simulink model "sevietta_devel_2017j"  (R2013a)
(part 3 of 32)

      | %     if length(current_widths) ~= numios,
      | %         error('%d field names specified, but %d widths?', numios, length(current_widths));
      | %     end
      | % end
      | % total_width = 0;
      | % for ctr = 1 : length(current_widths),
      | %     total_width = total_width + current_widths(ctr);
      | % end
      | % if total_width > 32,
      | %     error('Total width must be 32 or less, set to %d.', total_width);
      | % end
      mask Callback arith_types:
      | [numios, ~, ~, ~, current_types] = swreg_maskcheck(gcb);
      | % blk = gcb;
      | % mode = get_param(blk, 'mode');
      | % current_types = eval(get_param(blk, 'arith_types'));
      | % numios = length(current_types);
      | % if (strcmp(mode, 'one value') || strcmp(mode, 'fields of equal size')) && (length(current_types) > 1),
      | %     error('Only one type may be specified for this mode.');
      | % elseif strcmp(mode, 'fields of arbitrary size')
      | %     current_names = textscan(strtrim(strrep(strrep(get_param(blk, 'names'), ']', ''), '[', '')), '%s');
      | %     current_names = current_names{1};
      | %     numios = length(current_names);
      | %     if length(current_types) ~= numios,
      | %         error('%d field names specified, but %d types?', numios, length(current_types));
      | %     end
      | % end
      | problem = 0;
      | for ctr = 1 : numios,
      |     t = current_types(ctr);
      |     if (t < 0) || (t > 2),
      |         problem = t;
      |         ctr = numios + 1;
      |     end
      | end
      | if problem ~= 0,
      |     error('Type cannot be %i, must be 0, 1 or 2.', problem);
      | end
      mask Callback bin_pts:
      | swreg_maskcheck(gcb);
      | % blk = gcb;
      | % mode = get_param(blk, 'mode');
      | % current_bins = eval(get_param(blk, 'bin_pts'));
      | % if (strcmp(mode, 'one value') || strcmp(mode, 'fields of equal size')) && (length(current_bins) > 1),
      | %     error('Only one binary pt may be specified for this mode.');
      | % elseif strcmp(mode, 'fields of arbitrary size')
      | %     current_names = textscan(strtrim(strrep(strrep(get_param(blk, 'names'), ']', ''), '[', '')), '%s');
      | %     current_names = current_names{1};
      | %     numios = length(current_names);
      | %     if length(current_bins) ~= numios,
      | %         error('%d field names specified, but %d binary pts?', numios, length(current_bins));
      | %     end
      | % end
  edge_detect1 : Subsystem  AncestorBlock=casper_library_misc/edge_detect  mask(edge_detect){edge=Rising, polarity=Active High, x_in=[0 0.08 0.08 0.16 0.16 0.24 0.24 0.32 0.32 0.4], y_in=[-1 -1  1  1  1  1  1  1  1  1], x_out=[0.6 0.68 0.68 0.76 0.76 0.84 0.84 0.92 0.92 1], y_out=[-1 -1  1  1 -1 -1 -1 -1 -1 -1]}
      mask prompts: edge "Edge Type"; polarity "Output Polarity"; x_in "Input X Positions"; y_in "Input Y Positions"; x_out "Output X Positions"; y_out "Output Y Positions"
      mask help: Output is active for one-cycle after each edge of the specified type (i.e. rising, falling or both).
      mask init:
      | edge_detect_init(gcb,...
      |     'edge',edge,...
      |     'polarity',polarity,...
      |     'x_in',x_in,...
      |     'x_out',x_out,...
      |     'y_in',y_in,...
      |     'y_out',y_out);
      | 
      | x_in_num=str2num(getfield(getfield(get_param(gcb,'UserData'),'parameters'),'x_in'));
      | x_out_num=str2num(getfield(getfield(get_param(gcb,'UserData'),'parameters'),'x_out'));
      | y_in_num=str2num(getfield(getfield(get_param(gcb,'UserData'),'parameters'),'y_in'));
      | y_out_num=str2num(getfield(getfield(get_param(gcb,'UserData'),'parameters'),'y_out'));
      settings: AttributesFormatString=|
      | rising edges
      | active high
      mask Help: Output is active for one-cycle after each edge of the specified type (i.e. rising, falling, or both).  Latency is zero.
      mask TypeOptions edge: Rising | Falling | Both
      mask TypeOptions polarity: Active High | Active Low
      mask Display:
      | plot(x_in_num,0.5+y_in_num*0.2);
      | plot(x_out_num,0.5+y_out_num*0.2);
  edge_detect2 : Subsystem  AncestorBlock=casper_library_misc/edge_detect  mask(edge_detect){edge=Rising, polarity=Active High, x_in=[0 0.08 0.08 0.16 0.16 0.24 0.24 0.32 0.32 0.4], y_in=[-1 -1  1  1  1  1  1  1  1  1], x_out=[0.6 0.68 0.68 0.76 0.76 0.84 0.84 0.92 0.92 1], y_out=[-1 -1  1  1 -1 -1 -1 -1 -1 -1]}
      mask prompts: edge "Edge Type"; polarity "Output Polarity"; x_in "Input X Positions"; y_in "Input Y Positions"; x_out "Output X Positions"; y_out "Output Y Positions"
      mask help: Output is active for one-cycle after each edge of the specified type (i.e. rising, falling or both).
      mask init: same as sevietta_devel_2017j/adc/edge_detect1
      settings: AttributesFormatString=|
      | rising edges
      | active high
      mask Help: Output is active for one-cycle after each edge of the specified type (i.e. rising, falling, or both).  Latency is zero.
      mask TypeOptions edge: Rising | Falling | Both
      mask TypeOptions polarity: Active High | Active Low
      mask Display:
      | plot(x_in_num,0.5+y_in_num*0.2);
      | plot(x_out_num,0.5+y_out_num*0.2);
  err_clear_sim{1..33} (33 alike) : Constant  Value=0
  force_sync : Subsystem  Tag=xps:sw_reg  AncestorBlock=xps_library/software_register  mask(swreg){mode=one value, io_dir=From Processor, io_delay=0, sample_period=1, names=reg, bitwidths=32, arith_types=0, bin_pts=0, sim_port=on, show_format=off}
      mask prompts: io_dir "I/O direction"; io_delay "I/O delay"; sample_period "Sample period"; names "Name:"; bitwidths "Bitwidth:"; arith_types "Type (ufix=0, fix=1, bool=2):"; bin_pts "Binary pt:"; sim_port "Provide sim input/output?"; show_format "Print format string?"
      mask init:
      | swreg_init(gcb)
      settings: AttributesFormatString=1input
      mask TypeOptions mode: one value | fields of equal size | fields of arbitrary size
      mask Callback mode: swreg_cb(gcb);
      mask TypeOptions io_dir: To Processor | From Processor
      mask Callback io_dir:
      | mask_enables = get_param(gcb, 'MaskEnables');
      | mask_names = get_param(gcb, 'MaskNames');
      | if strcmp(get_param(gcb, 'io_dir'), 'To Processor'),
      |     mask_enables{ismember(mask_names, 'sample_period')} = 'off';
      | else
      |     mask_enables{ismember(mask_names, 'sample_period')} = 'on';
      | end
      | set_param(gcb, 'MaskEnables', mask_enables);
      mask Callback bitwidths:
      | swreg_maskcheck(gcb);
      | % blk = gcb;
      | % mode = get_param(blk, 'mode');
      | % current_widths = eval(get_param(blk, 'bitwidths'));
      | % if (strcmp(mode, 'one value') || strcmp(mode, 'fields of equal size')) && (length(current_widths) > 1),
      | %     error('Only one width may be specified for this mode.');
      | % elseif strcmp(mode, 'fields of arbitrary size')
      | %     current_names = textscan(strtrim(strrep(strrep(get_param(blk, 'names'), ']', ''), '[', '')), '%s');
      | %     current_names = current_names{1};
      | %     numios = length(current_names);
      | %     if length(current_widths) ~= numios,
      | %         error('%d field names specified, but %d widths?', numios, length(current_widths));
      | %     end
      | % end
      | % total_width = 0;
      | % for ctr = 1 : length(current_widths),
      | %     total_width = total_width + current_widths(ctr);
      | % end
      | % if total_width > 32,
      | %     error('Total width must be 32 or less, set to %d.', total_width);
      | % end
      mask Callback arith_types:
      | [numios, ~, ~, ~, current_types] = swreg_maskcheck(gcb);
      | % blk = gcb;
      | % mode = get_param(blk, 'mode');
      | % current_types = eval(get_param(blk, 'arith_types'));
      | % numios = length(current_types);
      | % if (strcmp(mode, 'one value') || strcmp(mode, 'fields of equal size')) && (length(current_types) > 1),
      | %     error('Only one type may be specified for this mode.');
      | % elseif strcmp(mode, 'fields of arbitrary size')
      | %     current_names = textscan(strtrim(strrep(strrep(get_param(blk, 'names'), ']', ''), '[', '')), '%s');
      | %     current_names = current_names{1};
      | %     numios = length(current_names);
      | %     if length(current_types) ~= numios,
      | %         error('%d field names specified, but %d types?', numios, length(current_types));
      | %     end
      | % end
      | problem = 0;
      | for ctr = 1 : numios,
      |     t = current_types(ctr);
      |     if (t < 0) || (t > 2),
      |         problem = t;
      |         ctr = numios + 1;
      |     end
      | end
      | if problem ~= 0,
      |     error('Type cannot be %i, must be 0, 1 or 2.', problem);
      | end
      mask Callback bin_pts:
      | swreg_maskcheck(gcb);
      | % blk = gcb;
      | % mode = get_param(blk, 'mode');
      | % current_bins = eval(get_param(blk, 'bin_pts'));
      | % if (strcmp(mode, 'one value') || strcmp(mode, 'fields of equal size')) && (length(current_bins) > 1),
      | %     error('Only one binary pt may be specified for this mode.');
      | % elseif strcmp(mode, 'fields of arbitrary size')
      | %     current_names = textscan(strtrim(strrep(strrep(get_param(blk, 'names'), ']', ''), '[', '')), '%s');
      | %     current_names = current_names{1};
      | %     numios = length(current_names);
      | %     if length(current_bins) ~= numios,
      | %         error('%d field names specified, but %d binary pts?', numios, length(current_bins));
      | %     end
      | % end
  led_pps : xps_library/gpio  Tag=xps:gpio  io_group=ROACH2:gpio  io_dir=out  arith_type=Boolean  bitwidth=1  bin_pt=0  bit_index=0  sample_period=1  use_single_ended=off  use_ddr=off  reg_iob=on  reg_clk_phase=0  termination=None
  led_tx : xps_library/gpio  Tag=xps:gpio  io_group=ROACH2:gpio  io_dir=out  arith_type=Boolean  bitwidth=1  bin_pt=0  bit_index=1  sample_period=1  use_single_ended=off  use_ddr=off  reg_iob=on  reg_clk_phase=0  termination=None
  pipeline33 : Subsystem  AncestorBlock=casper_library_delays/pipeline  mask(pipeline){latency=1}
      mask help:
      | An explicitly laid-out delay line to avoid mapping to SRL16s
      | for use in pipelining to help achieve timing closure.
      mask init:
      | pipeline_init(gcb,'latency',latency);
      settings: AttributesFormatString=Latency = %<latency>
      mask Display:
      | port_label('input', 1, 'd');
      | port_label('output', 1, 'q');
      | disp(['Z^-', num2str(latency)]);
  pipeline34 : Subsystem  AncestorBlock=casper_library_delays/pipeline  mask(pipeline){latency=1}
      mask help:
      | An explicitly laid-out delay line to avoid mapping to SRL16s
      | for use in pipelining to help achieve timing closure.
      mask init:
      | pipeline_init(gcb,'latency',latency);
      settings: AttributesFormatString=Latency = %<latency>
      mask Display:
      | port_label('input', 1, 'd');
      | port_label('output', 1, 'q');
      | disp(['Z^-', num2str(latency)]);
  pipeline35 : Subsystem  AncestorBlock=casper_library_delays/pipeline  mask(pipeline){latency=1}
      mask help:
      | An explicitly laid-out delay line to avoid mapping to SRL16s
      | for use in pipelining to help achieve timing closure.
      mask init:
      | pipeline_init(gcb,'latency',latency);
      settings: AttributesFormatString=Latency = %<latency>
      mask Display:
      | port_label('input', 1, 'd');
      | port_label('output', 1, 'q');
      | disp(['Z^-', num2str(latency)]);
  pipeline36 : Subsystem  AncestorBlock=casper_library_delays/pipeline  mask(pipeline){latency=1}
      mask help:
      | An explicitly laid-out delay line to avoid mapping to SRL16s
      | for use in pipelining to help achieve timing closure.
      mask init:
      | pipeline_init(gcb,'latency',latency);
      settings: AttributesFormatString=Latency = %<latency>
      mask Display:
      | port_label('input', 1, 'd');
      | port_label('output', 1, 'q');
      | disp(['Z^-', num2str(latency)]);
  pipeline37 : Subsystem  AncestorBlock=casper_library_delays/pipeline  mask(pipeline){latency=1}
      mask help:
      | An explicitly laid-out delay line to avoid mapping to SRL16s
      | for use in pipelining to help achieve timing closure.
      mask init:
      | pipeline_init(gcb,'latency',latency);
      settings: AttributesFormatString=Latency = %<latency>
      mask Display:
      | port_label('input', 1, 'd');
      | port_label('output', 1, 'q');
      | disp(['Z^-', num2str(latency)]);
  pipeline38 : Subsystem  AncestorBlock=casper_library_delays/pipeline  mask(pipeline){latency=1}
      mask help:
      | An explicitly laid-out delay line to avoid mapping to SRL16s
      | for use in pipelining to help achieve timing closure.
      mask init:
      | pipeline_init(gcb,'latency',latency);
      settings: AttributesFormatString=Latency = %<latency>
      mask Display:
      | port_label('input', 1, 'd');
      | port_label('output', 1, 'q');
      | disp(['Z^-', num2str(latency)]);
  pipeline39 : Subsystem  AncestorBlock=casper_library_delays/pipeline  mask(pipeline){latency=1}
      mask help:
      | An explicitly laid-out delay line to avoid mapping to SRL16s
      | for use in pipelining to help achieve timing closure.
      mask init:
      | pipeline_init(gcb,'latency',latency);
      settings: AttributesFormatString=Latency = %<latency>
      mask Display:
      | port_label('input', 1, 'd');
      | port_label('output', 1, 'q');
      | disp(['Z^-', num2str(latency)]);
  pipeline40 : Subsystem  AncestorBlock=casper_library_delays/pipeline  mask(pipeline){latency=1}
      mask help:
      | An explicitly laid-out delay line to avoid mapping to SRL16s
      | for use in pipelining to help achieve timing closure.
      mask init:
      | pipeline_init(gcb,'latency',latency);
      settings: AttributesFormatString=Latency = %<latency>
      mask Display:
      | port_label('input', 1, 'd');
      | port_label('output', 1, 'q');
      | disp(['Z^-', num2str(latency)]);
  pipeline41 : Subsystem  AncestorBlock=casper_library_delays/pipeline  mask(pipeline){latency=1}
      mask help:
      | An explicitly laid-out delay line to avoid mapping to SRL16s
      | for use in pipelining to help achieve timing closure.
      mask init:
      | pipeline_init(gcb,'latency',latency);
      settings: AttributesFormatString=Latency = %<latency>
      mask Display:
      | port_label('input', 1, 'd');
      | port_label('output', 1, 'q');
      | disp(['Z^-', num2str(latency)]);
  pipeline42 : Subsystem  AncestorBlock=casper_library_delays/pipeline  mask(pipeline){latency=1}
      mask help:
      | An explicitly laid-out delay line to avoid mapping to SRL16s
      | for use in pipelining to help achieve timing closure.
      mask init:
      | pipeline_init(gcb,'latency',latency);
      settings: AttributesFormatString=Latency = %<latency>
      mask Display:
      | port_label('input', 1, 'd');
      | port_label('output', 1, 'q');
      | disp(['Z^-', num2str(latency)]);
  pipeline43 : Subsystem  AncestorBlock=casper_library_delays/pipeline  mask(pipeline){latency=1}
      mask help:
      | An explicitly laid-out delay line to avoid mapping to SRL16s
      | for use in pipelining to help achieve timing closure.
      mask init:
      | pipeline_init(gcb,'latency',latency);
      settings: AttributesFormatString=Latency = %<latency>
      mask Display:
      | port_label('input', 1, 'd');
      | port_label('output', 1, 'q');
      | disp(['Z^-', num2str(latency)]);
  pipeline44 : Subsystem  AncestorBlock=casper_library_delays/pipeline  mask(pipeline){latency=1}
      mask help:
      | An explicitly laid-out delay line to avoid mapping to SRL16s
      | for use in pipelining to help achieve timing closure.
      mask init:
      | pipeline_init(gcb,'latency',latency);
      settings: AttributesFormatString=Latency = %<latency>
      mask Display:
      | port_label('input', 1, 'd');
      | port_label('output', 1, 'q');
      | disp(['Z^-', num2str(latency)]);
  pipeline45 : Subsystem  AncestorBlock=casper_library_delays/pipeline  mask(pipeline){latency=1}
      mask help:
      | An explicitly laid-out delay line to avoid mapping to SRL16s
      | for use in pipelining to help achieve timing closure.
      mask init:
      | pipeline_init(gcb,'latency',latency);
      settings: AttributesFormatString=Latency = %<latency>
      mask Display:
      | port_label('input', 1, 'd');
      | port_label('output', 1, 'q');
      | disp(['Z^-', num2str(latency)]);
  pipeline46 : Subsystem  AncestorBlock=casper_library_delays/pipeline  mask(pipeline){latency=1}
      mask help:
      | An explicitly laid-out delay line to avoid mapping to SRL16s
      | for use in pipelining to help achieve timing closure.
      mask init:
      | pipeline_init(gcb,'latency',latency);
      settings: AttributesFormatString=Latency = %<latency>
      mask Display:
      | port_label('input', 1, 'd');
      | port_label('output', 1, 'q');
      | disp(['Z^-', num2str(latency)]);
  pipeline47 : Subsystem  AncestorBlock=casper_library_delays/pipeline  mask(pipeline){latency=1}
      mask help:
      | An explicitly laid-out delay line to avoid mapping to SRL16s
      | for use in pipelining to help achieve timing closure.
      mask init:
      | pipeline_init(gcb,'latency',latency);
      settings: AttributesFormatString=Latency = %<latency>
      mask Display:
      | port_label('input', 1, 'd');
      | port_label('output', 1, 'q');
      | disp(['Z^-', num2str(latency)]);
  pipeline48 : Subsystem  AncestorBlock=casper_library_delays/pipeline  mask(pipeline){latency=1}
      mask help:
      | An explicitly laid-out delay line to avoid mapping to SRL16s
      | for use in pipelining to help achieve timing closure.
      mask init:
      | pipeline_init(gcb,'latency',latency);
      settings: AttributesFormatString=Latency = %<latency>
      mask Display:
      | port_label('input', 1, 'd');
      | port_label('output', 1, 'q');
      | disp(['Z^-', num2str(latency)]);
  pipeline49 : Subsystem  AncestorBlock=casper_library_delays/pipeline  mask(pipeline){latency=1}
      mask help:
      | An explicitly laid-out delay line to avoid mapping to SRL16s
      | for use in pipelining to help achieve timing closure.
      mask init:
      | pipeline_init(gcb,'latency',latency);
      settings: AttributesFormatString=Latency = %<latency>
      mask Display:
      | port_label('input', 1, 'd');
      | port_label('output', 1, 'q');
      | disp(['Z^-', num2str(latency)]);
  pipeline50 : Subsystem  AncestorBlock=casper_library_delays/pipeline  mask(pipeline){latency=1}
      mask help:
      | An explicitly laid-out delay line to avoid mapping to SRL16s
      | for use in pipelining to help achieve timing closure.
      mask init:
      | pipeline_init(gcb,'latency',latency);
      settings: AttributesFormatString=Latency = %<latency>
      mask Display:
      | port_label('input', 1, 'd');
      | port_label('output', 1, 'q');
      | disp(['Z^-', num2str(latency)]);
  pipeline51 : Subsystem  AncestorBlock=casper_library_delays/pipeline  mask(pipeline){latency=1}
      mask help:
      | An explicitly laid-out delay line to avoid mapping to SRL16s
      | for use in pipelining to help achieve timing closure.
      mask init:
      | pipeline_init(gcb,'latency',latency);
      settings: AttributesFormatString=Latency = %<latency>
      mask Display:
      | port_label('input', 1, 'd');
      | port_label('output', 1, 'q');
      | disp(['Z^-', num2str(latency)]);
  pipeline52 : Subsystem  AncestorBlock=casper_library_delays/pipeline  mask(pipeline){latency=1}
      mask help:
      | An explicitly laid-out delay line to avoid mapping to SRL16s
      | for use in pipelining to help achieve timing closure.
      mask init:
      | pipeline_init(gcb,'latency',latency);
      settings: AttributesFormatString=Latency = %<latency>
      mask Display:
      | port_label('input', 1, 'd');
      | port_label('output', 1, 'q');
      | disp(['Z^-', num2str(latency)]);
  pipeline53 : Subsystem  AncestorBlock=casper_library_delays/pipeline  mask(pipeline){latency=1}
      mask help:
      | An explicitly laid-out delay line to avoid mapping to SRL16s
      | for use in pipelining to help achieve timing closure.
      mask init:
      | pipeline_init(gcb,'latency',latency);
      settings: AttributesFormatString=Latency = %<latency>
      mask Display:
      | port_label('input', 1, 'd');
      | port_label('output', 1, 'q');
      | disp(['Z^-', num2str(latency)]);
  pipeline54 : Subsystem  AncestorBlock=casper_library_delays/pipeline  mask(pipeline){latency=1}
      mask help:
      | An explicitly laid-out delay line to avoid mapping to SRL16s
      | for use in pipelining to help achieve timing closure.
      mask init:
      | pipeline_init(gcb,'latency',latency);
      settings: AttributesFormatString=Latency = %<latency>
      mask Display:
      | port_label('input', 1, 'd');
      | port_label('output', 1, 'q');
      | disp(['Z^-', num2str(latency)]);
  pipeline55 : Subsystem  AncestorBlock=casper_library_delays/pipeline  mask(pipeline){latency=1}
      mask help:
      | An explicitly laid-out delay line to avoid mapping to SRL16s
      | for use in pipelining to help achieve timing closure.
      mask init:
      | pipeline_init(gcb,'latency',latency);
      settings: AttributesFormatString=Latency = %<latency>
      mask Display:
      | port_label('input', 1, 'd');
      | port_label('output', 1, 'q');
      | disp(['Z^-', num2str(latency)]);
  pipeline56 : Subsystem  AncestorBlock=casper_library_delays/pipeline  mask(pipeline){latency=1}
      mask help:
      | An explicitly laid-out delay line to avoid mapping to SRL16s
      | for use in pipelining to help achieve timing closure.
      mask init:
      | pipeline_init(gcb,'latency',latency);
      settings: AttributesFormatString=Latency = %<latency>
      mask Display:
      | port_label('input', 1, 'd');
      | port_label('output', 1, 'q');
      | disp(['Z^-', num2str(latency)]);
  pipeline57 : Subsystem  AncestorBlock=casper_library_delays/pipeline  mask(pipeline){latency=1}
      mask help:
      | An explicitly laid-out delay line to avoid mapping to SRL16s
      | for use in pipelining to help achieve timing closure.
      mask init:
      | pipeline_init(gcb,'latency',latency);
      settings: AttributesFormatString=Latency = %<latency>
      mask Display:
      | port_label('input', 1, 'd');
      | port_label('output', 1, 'q');
      | disp(['Z^-', num2str(latency)]);
  pipeline58 : Subsystem  AncestorBlock=casper_library_delays/pipeline  mask(pipeline){latency=1}
      mask help:
      | An explicitly laid-out delay line to avoid mapping to SRL16s
      | for use in pipelining to help achieve timing closure.
      mask init:
      | pipeline_init(gcb,'latency',latency);
      settings: AttributesFormatString=Latency = %<latency>
      mask Display:
      | port_label('input', 1, 'd');
      | port_label('output', 1, 'q');
      | disp(['Z^-', num2str(latency)]);
  pipeline59 : Subsystem  AncestorBlock=casper_library_delays/pipeline  mask(pipeline){latency=1}
      mask help:
      | An explicitly laid-out delay line to avoid mapping to SRL16s
      | for use in pipelining to help achieve timing closure.
      mask init:
      | pipeline_init(gcb,'latency',latency);
      settings: AttributesFormatString=Latency = %<latency>
      mask Display:
      | port_label('input', 1, 'd');
      | port_label('output', 1, 'q');
      | disp(['Z^-', num2str(latency)]);
  pipeline60 : Subsystem  AncestorBlock=casper_library_delays/pipeline  mask(pipeline){latency=1}
      mask help:
      | An explicitly laid-out delay line to avoid mapping to SRL16s
      | for use in pipelining to help achieve timing closure.
      mask init:
      | pipeline_init(gcb,'latency',latency);
      settings: AttributesFormatString=Latency = %<latency>
      mask Display:
      | port_label('input', 1, 'd');
      | port_label('output', 1, 'q');
      | disp(['Z^-', num2str(latency)]);
  pipeline61 : Subsystem  AncestorBlock=casper_library_delays/pipeline  mask(pipeline){latency=1}
      mask help:
      | An explicitly laid-out delay line to avoid mapping to SRL16s
      | for use in pipelining to help achieve timing closure.
      mask init:
      | pipeline_init(gcb,'latency',latency);
      settings: AttributesFormatString=Latency = %<latency>
      mask Display:
      | port_label('input', 1, 'd');
      | port_label('output', 1, 'q');
      | disp(['Z^-', num2str(latency)]);
  pipeline62 : Subsystem  AncestorBlock=casper_library_delays/pipeline  mask(pipeline){latency=1}
      mask help:
      | An explicitly laid-out delay line to avoid mapping to SRL16s
      | for use in pipelining to help achieve timing closure.
      mask init:
      | pipeline_init(gcb,'latency',latency);
      settings: AttributesFormatString=Latency = %<latency>
      mask Display:
      | port_label('input', 1, 'd');
      | port_label('output', 1, 'q');
      | disp(['Z^-', num2str(latency)]);
  pipeline63 : Subsystem  AncestorBlock=casper_library_delays/pipeline  mask(pipeline){latency=1}
      mask help:
      | An explicitly laid-out delay line to avoid mapping to SRL16s
      | for use in pipelining to help achieve timing closure.
      mask init:
      | pipeline_init(gcb,'latency',latency);
      settings: AttributesFormatString=Latency = %<latency>
      mask Display:
      | port_label('input', 1, 'd');
      | port_label('output', 1, 'q');
      | disp(['Z^-', num2str(latency)]);
  pipeline64 : Subsystem  AncestorBlock=casper_library_delays/pipeline  mask(pipeline){latency=1}
      mask help:
      | An explicitly laid-out delay line to avoid mapping to SRL16s
      | for use in pipelining to help achieve timing closure.
      mask init:
      | pipeline_init(gcb,'latency',latency);
      settings: AttributesFormatString=Latency = %<latency>
      mask Display:
      | port_label('input', 1, 'd');
      | port_label('output', 1, 'q');
      | disp(['Z^-', num2str(latency)]);
  pipeline65 : Subsystem  AncestorBlock=casper_library_delays/pipeline  mask(pipeline){latency=1}
      mask help:
      | An explicitly laid-out delay line to avoid mapping to SRL16s
      | for use in pipelining to help achieve timing closure.
      mask init:
      | pipeline_init(gcb,'latency',latency);
      settings: AttributesFormatString=Latency = %<latency>
      mask Display:
      | port_label('input', 1, 'd');
      | port_label('output', 1, 'q');
      | disp(['Z^-', num2str(latency)]);
  pipeline66 : Subsystem  AncestorBlock=casper_library_delays/pipeline  mask(pipeline){latency=1}
      mask help:
      | An explicitly laid-out delay line to avoid mapping to SRL16s
      | for use in pipelining to help achieve timing closure.
      mask init:
      | pipeline_init(gcb,'latency',latency);
      settings: AttributesFormatString=Latency = %<latency>
      mask Display:
      | port_label('input', 1, 'd');
      | port_label('output', 1, 'q');
      | disp(['Z^-', num2str(latency)]);
  pipeline67 : Subsystem  AncestorBlock=casper_library_delays/pipeline  mask(pipeline){latency=1}
      mask help:
      | An explicitly laid-out delay line to avoid mapping to SRL16s
      | for use in pipelining to help achieve timing closure.
      mask init:
      | pipeline_init(gcb,'latency',latency);
      settings: AttributesFormatString=Latency = %<latency>
      mask Display:
      | port_label('input', 1, 'd');
      | port_label('output', 1, 'q');
      | disp(['Z^-', num2str(latency)]);
  pipeline68 : Subsystem  AncestorBlock=casper_library_delays/pipeline  mask(pipeline){latency=1}
      mask help:
      | An explicitly laid-out delay line to avoid mapping to SRL16s
      | for use in pipelining to help achieve timing closure.
      mask init:
      | pipeline_init(gcb,'latency',latency);
      settings: AttributesFormatString=Latency = %<latency>
      mask Display:
      | port_label('input', 1, 'd');
      | port_label('output', 1, 'q');
      | disp(['Z^-', num2str(latency)]);
  pipeline69 : Subsystem  AncestorBlock=casper_library_delays/pipeline  mask(pipeline){latency=1}
      mask help:
      | An explicitly laid-out delay line to avoid mapping to SRL16s
      | for use in pipelining to help achieve timing closure.
      mask init:
      | pipeline_init(gcb,'latency',latency);
      settings: AttributesFormatString=Latency = %<latency>
      mask Display:
      | port_label('input', 1, 'd');
      | port_label('output', 1, 'q');
      | disp(['Z^-', num2str(latency)]);
  pipeline70 : Subsystem  AncestorBlock=casper_library_delays/pipeline  mask(pipeline){latency=1}
      mask help:
      | An explicitly laid-out delay line to avoid mapping to SRL16s
      | for use in pipelining to help achieve timing closure.
      mask init:
      | pipeline_init(gcb,'latency',latency);
      settings: AttributesFormatString=Latency = %<latency>
      mask Display:
      | port_label('input', 1, 'd');
      | port_label('output', 1, 'q');
      | disp(['Z^-', num2str(latency)]);
  pipeline71 : Subsystem  AncestorBlock=casper_library_delays/pipeline  mask(pipeline){latency=1}
      mask help:
      | An explicitly laid-out delay line to avoid mapping to SRL16s
      | for use in pipelining to help achieve timing closure.
      mask init:
      | pipeline_init(gcb,'latency',latency);
      settings: AttributesFormatString=Latency = %<latency>
      mask Display:
      | port_label('input', 1, 'd');
      | port_label('output', 1, 'q');
      | disp(['Z^-', num2str(latency)]);
  pipeline72 : Subsystem  AncestorBlock=casper_library_delays/pipeline  mask(pipeline){latency=1}
      mask help:
      | An explicitly laid-out delay line to avoid mapping to SRL16s
      | for use in pipelining to help achieve timing closure.
      mask init:
      | pipeline_init(gcb,'latency',latency);
      settings: AttributesFormatString=Latency = %<latency>
      mask Display:
      | port_label('input', 1, 'd');
      | port_label('output', 1, 'q');
      | disp(['Z^-', num2str(latency)]);
  pipeline73 : Subsystem  AncestorBlock=casper_library_delays/pipeline  mask(pipeline){latency=1}
      mask help:
      | An explicitly laid-out delay line to avoid mapping to SRL16s
      | for use in pipelining to help achieve timing closure.
      mask init:
      | pipeline_init(gcb,'latency',latency);
      settings: AttributesFormatString=Latency = %<latency>
      mask Display:
      | port_label('input', 1, 'd');
      | port_label('output', 1, 'q');
      | disp(['Z^-', num2str(latency)]);
  pulse_ext3 : casper_library_misc/pulse_ext  pulse_len=2^24
  rst : Subsystem  Tag=xps:sw_reg  AncestorBlock=xps_library/software_register  mask(swreg){mode=one value, io_dir=From Processor, io_delay=0, sample_period=1, names=reg, bitwidths=32, arith_types=0, bin_pts=0, sim_port=on, show_format=off}
      mask prompts: io_dir "I/O direction"; io_delay "I/O delay"; sample_period "Sample period"; names "Name:"; bitwidths "Bitwidth:"; arith_types "Type (ufix=0, fix=1, bool=2):"; bin_pts "Binary pt:"; sim_port "Provide sim input/output?"; show_format "Print format string?"
      mask init:
      | swreg_init(gcb)
      settings: AttributesFormatString=1input
      mask TypeOptions mode: one value | fields of equal size | fields of arbitrary size
      mask Callback mode: swreg_cb(gcb);
      mask TypeOptions io_dir: To Processor | From Processor
      mask Callback io_dir:
      | mask_enables = get_param(gcb, 'MaskEnables');
      | mask_names = get_param(gcb, 'MaskNames');
      | if strcmp(get_param(gcb, 'io_dir'), 'To Processor'),
      |     mask_enables{ismember(mask_names, 'sample_period')} = 'off';
      | else
      |     mask_enables{ismember(mask_names, 'sample_period')} = 'on';
      | end
      | set_param(gcb, 'MaskEnables', mask_enables);
      mask Callback bitwidths:
      | swreg_maskcheck(gcb);
      | % blk = gcb;
      | % mode = get_param(blk, 'mode');
      | % current_widths = eval(get_param(blk, 'bitwidths'));
      | % if (strcmp(mode, 'one value') || strcmp(mode, 'fields of equal size')) && (length(current_widths) > 1),
      | %     error('Only one width may be specified for this mode.');
      | % elseif strcmp(mode, 'fields of arbitrary size')
      | %     current_names = textscan(strtrim(strrep(strrep(get_param(blk, 'names'), ']', ''), '[', '')), '%s');
      | %     current_names = current_names{1};
      | %     numios = length(current_names);
      | %     if length(current_widths) ~= numios,
      | %         error('%d field names specified, but %d widths?', numios, length(current_widths));
      | %     end
      | % end
      | % total_width = 0;
      | % for ctr = 1 : length(current_widths),
      | %     total_width = total_width + current_widths(ctr);
      | % end
      | % if total_width > 32,
      | %     error('Total width must be 32 or less, set to %d.', total_width);
      | % end
      mask Callback arith_types:
      | [numios, ~, ~, ~, current_types] = swreg_maskcheck(gcb);
      | % blk = gcb;
      | % mode = get_param(blk, 'mode');
      | % current_types = eval(get_param(blk, 'arith_types'));
      | % numios = length(current_types);
      | % if (strcmp(mode, 'one value') || strcmp(mode, 'fields of equal size')) && (length(current_types) > 1),
      | %     error('Only one type may be specified for this mode.');
      | % elseif strcmp(mode, 'fields of arbitrary size')
      | %     current_names = textscan(strtrim(strrep(strrep(get_param(blk, 'names'), ']', ''), '[', '')), '%s');
      | %     current_names = current_names{1};
      | %     numios = length(current_names);
      | %     if length(current_types) ~= numios,
      | %         error('%d field names specified, but %d types?', numios, length(current_types));
      | %     end
      | % end
      | problem = 0;
      | for ctr = 1 : numios,
      |     t = current_types(ctr);
      |     if (t < 0) || (t > 2),
      |         problem = t;
      |         ctr = numios + 1;
      |     end
      | end
      | if problem ~= 0,
      |     error('Type cannot be %i, must be 0, 1 or 2.', problem);
      | end
      mask Callback bin_pts:
      | swreg_maskcheck(gcb);
      | % blk = gcb;
      | % mode = get_param(blk, 'mode');
      | % current_bins = eval(get_param(blk, 'bin_pts'));
      | % if (strcmp(mode, 'one value') || strcmp(mode, 'fields of equal size')) && (length(current_bins) > 1),
      | %     error('Only one binary pt may be specified for this mode.');
      | % elseif strcmp(mode, 'fields of arbitrary size')
      | %     current_names = textscan(strtrim(strrep(strrep(get_param(blk, 'names'), ']', ''), '[', '')), '%s');
      | %     current_names = current_names{1};
      | %     numios = length(current_names);
      | %     if length(current_bins) ~= numios,
      | %         error('%d field names specified, but %d binary pts?', numios, length(current_bins));
      | %     end
      | % end
  sync_count : Subsystem  Tag=xps:sw_reg  AncestorBlock=xps_library/software_register  mask(swreg){mode=one value, io_dir=To Processor, io_delay=0, sample_period=1, names=reg, bitwidths=32, arith_types=0, bin_pts=0, sim_port=on, show_format=off}
      mask prompts: io_dir "I/O direction"; io_delay "I/O delay"; sample_period "Sample period"; names "Name:"; bitwidths "Bitwidth:"; arith_types "Type (ufix=0, fix=1, bool=2):"; bin_pts "Binary pt:"; sim_port "Provide sim input/output?"; show_format "Print format string?"
      mask init:
      | swreg_init(gcb)
      settings: AttributesFormatString=1output
      mask TypeOptions mode: one value | fields of equal size | fields of arbitrary size
      mask Callback mode: swreg_cb(gcb);
      mask TypeOptions io_dir: To Processor | From Processor
      mask Callback io_dir:
      | mask_enables = get_param(gcb, 'MaskEnables');
      | mask_names = get_param(gcb, 'MaskNames');
      | if strcmp(get_param(gcb, 'io_dir'), 'To Processor'),
      |     mask_enables{ismember(mask_names, 'sample_period')} = 'off';
      | else
      |     mask_enables{ismember(mask_names, 'sample_period')} = 'on';
      | end
      | set_param(gcb, 'MaskEnables', mask_enables);
      mask Callback bitwidths:
      | swreg_maskcheck(gcb);
      | % blk = gcb;
      | % mode = get_param(blk, 'mode');
      | % current_widths = eval(get_param(blk, 'bitwidths'));
      | % if (strcmp(mode, 'one value') || strcmp(mode, 'fields of equal size')) && (length(current_widths) > 1),
      | %     error('Only one width may be specified for this mode.');
      | % elseif strcmp(mode, 'fields of arbitrary size')
      | %     current_names = textscan(strtrim(strrep(strrep(get_param(blk, 'names'), ']', ''), '[', '')), '%s');
      | %     current_names = current_names{1};
      | %     numios = length(current_names);
      | %     if length(current_widths) ~= numios,
      | %         error('%d field names specified, but %d widths?', numios, length(current_widths));
      | %     end
      | % end
      | % total_width = 0;
      | % for ctr = 1 : length(current_widths),
      | %     total_width = total_width + current_widths(ctr);
      | % end
      | % if total_width > 32,
      | %     error('Total width must be 32 or less, set to %d.', total_width);
      | % end
      mask Callback arith_types:
      | [numios, ~, ~, ~, current_types] = swreg_maskcheck(gcb);
      | % blk = gcb;
      | % mode = get_param(blk, 'mode');
      | % current_types = eval(get_param(blk, 'arith_types'));
      | % numios = length(current_types);
      | % if (strcmp(mode, 'one value') || strcmp(mode, 'fields of equal size')) && (length(current_types) > 1),
      | %     error('Only one type may be specified for this mode.');
      | % elseif strcmp(mode, 'fields of arbitrary size')
      | %     current_names = textscan(strtrim(strrep(strrep(get_param(blk, 'names'), ']', ''), '[', '')), '%s');
      | %     current_names = current_names{1};
      | %     numios = length(current_names);
      | %     if length(current_types) ~= numios,
      | %         error('%d field names specified, but %d types?', numios, length(current_types));
      | %     end
      | % end
      | problem = 0;
      | for ctr = 1 : numios,
      |     t = current_types(ctr);
      |     if (t < 0) || (t > 2),
      |         problem = t;
      |         ctr = numios + 1;
      |     end
      | end
      | if problem ~= 0,
      |     error('Type cannot be %i, must be 0, 1 or 2.', problem);
      | end
      mask Callback bin_pts:
      | swreg_maskcheck(gcb);
      | % blk = gcb;
      | % mode = get_param(blk, 'mode');
      | % current_bins = eval(get_param(blk, 'bin_pts'));
      | % if (strcmp(mode, 'one value') || strcmp(mode, 'fields of equal size')) && (length(current_bins) > 1),
      | %     error('Only one binary pt may be specified for this mode.');
      | % elseif strcmp(mode, 'fields of arbitrary size')
      | %     current_names = textscan(strtrim(strrep(strrep(get_param(blk, 'names'), ']', ''), '[', '')), '%s');
      | %     current_names = current_names{1};
      | %     numios = length(current_names);
      | %     if length(current_bins) ~= numios,
      | %         error('%d field names specified, but %d binary pts?', numios, length(current_bins));
      | %     end
      | % end
  sync_in : xps_library/gpio  Tag=xps:gpio  io_group=ROACH2:sync_in  io_dir=in  arith_type=Boolean  bitwidth=1  bin_pt=0  bit_index=0  sample_period=1  use_single_ended=off  use_ddr=off  reg_iob=on  reg_clk_phase=0  termination=None
  sync_out : xps_library/gpio  Tag=xps:gpio  io_group=ROACH2:sync_out  io_dir=out  arith_type=Boolean  bitwidth=1  bin_pt=0  bit_index=0  sample_period=1  use_single_ended=off  use_ddr=off  reg_iob=on  reg_clk_phase=0  termination=None
  sync_pulse : Subsystem  Tag=xps:sw_reg  AncestorBlock=xps_library/software_register  mask(swreg){mode=one value, io_dir=To Processor, io_delay=0, sample_period=1, names=reg, bitwidths=32, arith_types=0, bin_pts=0, sim_port=on, show_format=off}
      mask prompts: io_dir "I/O direction"; io_delay "I/O delay"; sample_period "Sample period"; names "Name:"; bitwidths "Bitwidth:"; arith_types "Type (ufix=0, fix=1, bool=2):"; bin_pts "Binary pt:"; sim_port "Provide sim input/output?"; show_format "Print format string?"
      mask init:
      | swreg_init(gcb)
      settings: AttributesFormatString=1output
      mask TypeOptions mode: one value | fields of equal size | fields of arbitrary size
      mask Callback mode: swreg_cb(gcb);
      mask TypeOptions io_dir: To Processor | From Processor
      mask Callback io_dir:
      | mask_enables = get_param(gcb, 'MaskEnables');
      | mask_names = get_param(gcb, 'MaskNames');
      | if strcmp(get_param(gcb, 'io_dir'), 'To Processor'),
      |     mask_enables{ismember(mask_names, 'sample_period')} = 'off';
      | else
      |     mask_enables{ismember(mask_names, 'sample_period')} = 'on';
      | end
      | set_param(gcb, 'MaskEnables', mask_enables);
      mask Callback bitwidths:
      | swreg_maskcheck(gcb);
      | % blk = gcb;
      | % mode = get_param(blk, 'mode');
      | % current_widths = eval(get_param(blk, 'bitwidths'));
      | % if (strcmp(mode, 'one value') || strcmp(mode, 'fields of equal size')) && (length(current_widths) > 1),
      | %     error('Only one width may be specified for this mode.');
      | % elseif strcmp(mode, 'fields of arbitrary size')
      | %     current_names = textscan(strtrim(strrep(strrep(get_param(blk, 'names'), ']', ''), '[', '')), '%s');
      | %     current_names = current_names{1};
      | %     numios = length(current_names);
      | %     if length(current_widths) ~= numios,
      | %         error('%d field names specified, but %d widths?', numios, length(current_widths));
      | %     end
      | % end
      | % total_width = 0;
      | % for ctr = 1 : length(current_widths),
      | %     total_width = total_width + current_widths(ctr);
      | % end
      | % if total_width > 32,
      | %     error('Total width must be 32 or less, set to %d.', total_width);
      | % end
      mask Callback arith_types:
      | [numios, ~, ~, ~, current_types] = swreg_maskcheck(gcb);
      | % blk = gcb;
      | % mode = get_param(blk, 'mode');
      | % current_types = eval(get_param(blk, 'arith_types'));
      | % numios = length(current_types);
      | % if (strcmp(mode, 'one value') || strcmp(mode, 'fields of equal size')) && (length(current_types) > 1),
      | %     error('Only one type may be specified for this mode.');
      | % elseif strcmp(mode, 'fields of arbitrary size')
      | %     current_names = textscan(strtrim(strrep(strrep(get_param(blk, 'names'), ']', ''), '[', '')), '%s');
      | %     current_names = current_names{1};
      | %     numios = length(current_names);
      | %     if length(current_types) ~= numios,
      | %         error('%d field names specified, but %d types?', numios, length(current_types));
      | %     end
      | % end
      | problem = 0;
      | for ctr = 1 : numios,
      |     t = current_types(ctr);
      |     if (t < 0) || (t > 2),
      |         problem = t;
      |         ctr = numios + 1;
      |     end
      | end
      | if problem ~= 0,
      |     error('Type cannot be %i, must be 0, 1 or 2.', problem);
      | end
      mask Callback bin_pts:
      | swreg_maskcheck(gcb);
      | % blk = gcb;
      | % mode = get_param(blk, 'mode');
      | % current_bins = eval(get_param(blk, 'bin_pts'));
      | % if (strcmp(mode, 'one value') || strcmp(mode, 'fields of equal size')) && (length(current_bins) > 1),
      | %     error('Only one binary pt may be specified for this mode.');
      | % elseif strcmp(mode, 'fields of arbitrary size')
      | %     current_names = textscan(strtrim(strrep(strrep(get_param(blk, 'names'), ']', ''), '[', '')), '%s');
      | %     current_names = current_names{1};
      | %     numios = length(current_names);
      | %     if length(current_bins) ~= numios,
      | %         error('%d field names specified, but %d binary pts?', numios, length(current_bins));
      | %     end
      | % end
  system_counter1 : xbsIndex_r4/Counter  cnt_type=Free Running  cnt_to=Inf  operation=Up  start_count=0  cnt_by_val=1  arith_type=Unsigned  n_bits=32  bin_pt=0  load_pin=off  rst=on  en=on  explicit_period=on  period=1  dbl_ovrd=off  use_behavioral_HDL=off  implementation=Fabric  block_type=counter
      settings: block_version=11.4
  system_counter2 : xbsIndex_r4/Counter  cnt_type=Free Running  cnt_to=Inf  operation=Up  start_count=0  cnt_by_val=1  arith_type=Unsigned  n_bits=32  bin_pt=0  load_pin=off  rst=on  en=on  explicit_period=on  period=1  dbl_ovrd=off  use_behavioral_HDL=off  implementation=Fabric  block_type=counter
      settings: block_version=11.4
  ws0 : simulink/Sources/Repeating Sequence  rep_seq_t=v_time  rep_seq_y=v_pps
  Out2 : Outport
  tag scope: adc0=global, adc10=global, adc11=global, adc12=global, adc13=global, adc14=global, adc15=global, adc16=global, adc17=global, adc18=global, adc19=global, adc1=global, adc20=global, adc21=global, adc22=global, adc23=global, adc24=global, adc25=global, adc26=global, adc27=global, adc28=global, adc29=global, adc2=global, adc30=global, adc31=global, adc3=global, adc4=global, adc5=global, adc6=global, adc7=global, adc8=global, adc9=global, ain0=global, ain10=global, ain11=global, ain12=global, ain13=global, ain14=global, ain15=global, ain16=global, ain17=global, ain18=global, ain19=global, ain1=global, ain20=global, ain21=global, ain22=global, ain23=global, ain24=global, ain25=global, ain26=global, ain27=global, ain28=global, ain29=global, ain2=global, ain30=global, ain31=global, ain3=global, ain4=global, ain5=global, ain6=global, ain7=global, ain8=global, ain9=global, cnt_rst=global, core_rst=global, delay0=global, delay10=global, delay11=global, delay12=global, delay13=global, delay14=global, delay15=global, delay16=global, delay17=global, delay18=global, delay19=global, delay1=global, delay20=global, delay21=global, delay22=global, delay23=global, delay24=global, delay25=global, delay26=global, delay27=global, delay28=global, delay29=global, delay2=global, delay30=global, delay31=global, delay3=global, delay4=global, delay5=global, delay6=global, delay7=global, delay8=global, delay9=global, every_second=global, sync_pps=global, timing_sync=global
  wires:
  Counter Limited/1 -> adc16x250-8/1(a1_sim), adc16x250-8/2(a2_sim), adc16x250-8/3(a3_sim), adc16x250-8/4(a4_sim), adc16x250-8/5(b1_sim), adc16x250-8/6(b2_sim), adc16x250-8/7(b3_sim), adc16x250-8/8(b4_sim), adc16x250-8/9(c1_sim), adc16x250-8/10(c2_sim), adc16x250-8/11(c3_sim), adc16x250-8/12(c4_sim), adc16x250-8/13(d1_sim), adc16x250-8/14(d2_sim), adc16x250-8/15(d3_sim), adc16x250-8/16(d4_sim), adc16x250-8/17(e1_sim), adc16x250-8/18(e2_sim), adc16x250-8/19(e3_sim), adc16x250-8/20(e4_sim), adc16x250-8/21(f1_sim), adc16x250-8/22(f2_sim), adc16x250-8/23(f3_sim), adc16x250-8/24(f4_sim), adc16x250-8/25(g1_sim), adc16x250-8/26(g2_sim), adc16x250-8/27(g3_sim), adc16x250-8/28(g4_sim), adc16x250-8/29(h1_sim), adc16x250-8/30(h2_sim), adc16x250-8/32(h4_sim), adc16x250-8/31(h3_sim)
  Mux/1 -> Out2/1
  Constant2/1 -> Mux/1
  Constant3/1 -> Mux/2
  led_pps/1 -> Terminator5/1
  pipeline40/1(q) -> led_pps/1
  pulse_ext3/1 -> pipeline40/1(d)
  led_tx/1 -> Terminator7/1
  pipeline41/1(q) -> led_tx/1
  [led_tx] -> pipeline41/1(d)
  [sync_pps] -> pulse_ext3/1
  err_clear_sim5/1 -> rst/1(sim_1)
  rst/1(in_reg) -> pipeline34/1(d)
  Slice1/1 -> [cnt_rst]
  Slice3/1 -> [core_rst]
  force_sync/1(in_reg) -> pipeline35/1(d)
  Constant6/1 -> force_sync/1(sim_1)
  sync_out/1 -> Terminator1/1
  system_counter1/1 -> pipeline38/1(d), Relational3/1
  Constant10/1 -> Relational3/2
  [cnt_rst] -> system_counter1/1
  edge_detect1/1(out) -> pipeline45/1(d), system_counter1/2  "sync_rnd"
  Relational3/1 -> edge_detect2/1(in)
  edge_detect2/1(out) -> system_counter2/2, Logical1/2
  Slice4/1 -> Logical1/1, Terminator2/1
  sync_count/1(sim_out) -> Terminator3/1
  [cnt_rst] -> system_counter2/1
  system_counter2/1 -> pipeline36/1(d)
  sync_pulse/1(sim_out) -> Terminator4/1
  pipeline34/1(q) -> Slice3/1, Slice1/1
  pipeline35/1(q) -> Slice4/1
  pipeline36/1(q) -> sync_pulse/1(out_reg)
  pipeline37/1(q) -> sync_out/1
  pipeline38/1(q) -> sync_count/1(out_reg)
  pipeline45/1(q) -> [every_second], [sync_pps]
  ws0/1 -> sync_in/1
  sync_in/1 -> pipeline33/1(d)
  pipeline33/1(q) -> pipeline37/1(d), edge_detect1/1(in)
  err_clear_sim1/1 -> delay0/1(sim_1)
  delay0/1(in_reg) -> Slice/1
  err_clear_sim2/1 -> delay1/1(sim_1)
  delay1/1(in_reg) -> Slice2/1
  err_clear_sim3/1 -> delay2/1(sim_1)
  delay2/1(in_reg) -> Slice5/1
  err_clear_sim4/1 -> delay3/1(sim_1)
  delay3/1(in_reg) -> Slice6/1
  err_clear_sim6/1 -> delay4/1(sim_1)
  delay4/1(in_reg) -> Slice7/1
  err_clear_sim7/1 -> delay5/1(sim_1)
  delay5/1(in_reg) -> Slice8/1
  err_clear_sim8/1 -> delay6/1(sim_1)
  delay6/1(in_reg) -> Slice9/1
  err_clear_sim9/1 -> delay7/1(sim_1)
  delay7/1(in_reg) -> Slice10/1
  err_clear_sim10/1 -> delay8/1(sim_1)
  delay8/1(in_reg) -> Slice11/1
  err_clear_sim11/1 -> delay9/1(sim_1)
  delay9/1(in_reg) -> Slice13/1
  err_clear_sim12/1 -> delay10/1(sim_1)
  delay10/1(in_reg) -> Slice14/1
  err_clear_sim13/1 -> delay11/1(sim_1)
  delay11/1(in_reg) -> Slice15/1
  err_clear_sim14/1 -> delay12/1(sim_1)
  delay12/1(in_reg) -> Slice16/1
  err_clear_sim15/1 -> delay13/1(sim_1)
  delay13/1(in_reg) -> Slice17/1
  err_clear_sim16/1 -> delay14/1(sim_1)
  delay14/1(in_reg) -> Slice18/1
  err_clear_sim17/1 -> delay15/1(sim_1)
  delay15/1(in_reg) -> Slice12/1
  Slice/1 -> pipeline42/1(d)
  Slice2/1 -> pipeline43/1(d)
  Slice5/1 -> pipeline44/1(d)
  Slice6/1 -> pipeline46/1(d)
  Slice8/1 -> pipeline48/1(d)
  Slice7/1 -> pipeline47/1(d)
  Slice10/1 -> pipeline50/1(d)
  Slice9/1 -> pipeline49/1(d)
  Slice13/1 -> pipeline52/1(d)
  Slice12/1 -> pipeline58/1(d)
  Slice14/1 -> pipeline53/1(d)
  Slice17/1 -> pipeline56/1(d)
  Slice18/1 -> pipeline57/1(d)
  Slice11/1 -> pipeline51/1(d)
  Slice15/1 -> pipeline54/1(d)
  Slice16/1 -> pipeline55/1(d)
  coarse_delay/1(sync_out) -> [timing_sync]
  coarse_delay/2(out0) -> [adc0]
  coarse_delay/3(out1) -> [adc1]
  coarse_delay/6(out4) -> [adc4]
  coarse_delay/5(out3) -> [adc3]
  coarse_delay/7(out5) -> [adc5]
  coarse_delay/4(out2) -> [adc2]
  coarse_delay/8(out6) -> [adc6]
  coarse_delay/9(out7) -> [adc7]
  coarse_delay/10(out8) -> [adc8]
  coarse_delay/11(out9) -> [adc9]
  coarse_delay/12(out10) -> [adc10]
  coarse_delay/13(out11) -> [adc11]
  coarse_delay/14(out12) -> [adc12]
  coarse_delay/15(out13) -> [adc13]
  coarse_delay/16(out14) -> [adc14]
  coarse_delay/17(out15) -> [adc15]
  [sync_to_cdelay] -> coarse_delay/1(sync)
  [ain0] -> coarse_delay/3(in0)
  [delay0] -> coarse_delay/2(delay0)
  [ain1] -> coarse_delay/5(in1)
  [delay1] -> coarse_delay/4(delay1)
  [ain2] -> coarse_delay/7(in2)
  [delay2] -> coarse_delay/6(delay2)
  [ain3] -> coarse_delay/9(in3)
  [delay3] -> coarse_delay/8(delay3)
  [ain4] -> coarse_delay/11(in4)
  [delay4] -> coarse_delay/10(delay4)
  [ain5] -> coarse_delay/13(in5)
  [ain6] -> coarse_delay/15(in6)
  [ain7] -> coarse_delay/17(in7)
  [delay5] -> coarse_delay/12(delay5)
  [delay6] -> coarse_delay/14(delay6)
  [delay7] -> coarse_delay/16(delay7)
  [ain15] -> coarse_delay/33(in15)
  [ain10] -> coarse_delay/23(in10)
  [ain11] -> coarse_delay/25(in11)
  [ain12] -> coarse_delay/27(in12)
  [ain13] -> coarse_delay/29(in13)
  [ain14] -> coarse_delay/31(in14)
  [ain9] -> coarse_delay/21(in9)
  [ain8] -> coarse_delay/19(in8)
  [delay10] -> coarse_delay/22(delay10)
  [delay11] -> coarse_delay/24(delay11)
  [delay12] -> coarse_delay/26(delay12)
  [delay13] -> coarse_delay/28(delay13)
  [delay14] -> coarse_delay/30(delay14)
  [delay15] -> coarse_delay/32(delay15)
  [delay9] -> coarse_delay/20(delay9)
  [delay8] -> coarse_delay/18(delay8)
  err_clear_sim18/1 -> delay16/1(sim_1)
  delay16/1(in_reg) -> Slice19/1
  err_clear_sim27/1 -> delay17/1(sim_1)
  delay17/1(in_reg) -> Slice29/1
  err_clear_sim28/1 -> delay24/1(sim_1)
  delay24/1(in_reg) -> Slice30/1
  err_clear_sim29/1 -> delay25/1(sim_1)
  delay25/1(in_reg) -> Slice31/1
  err_clear_sim30/1 -> delay26/1(sim_1)
  delay26/1(in_reg) -> Slice32/1
  err_clear_sim31/1 -> delay27/1(sim_1)
  delay27/1(in_reg) -> Slice33/1
  err_clear_sim32/1 -> delay28/1(sim_1)
  delay28/1(in_reg) -> Slice34/1
  err_clear_sim33/1 -> delay29/1(sim_1)
  delay29/1(in_reg) -> Slice20/1
  err_clear_sim19/1 -> delay30/1(sim_1)
  delay30/1(in_reg) -> Slice21/1
  err_clear_sim20/1 -> delay31/1(sim_1)
  delay31/1(in_reg) -> Slice23/1
  err_clear_sim21/1 -> delay18/1(sim_1)
  delay18/1(in_reg) -> Slice24/1
  err_clear_sim22/1 -> delay19/1(sim_1)
  delay19/1(in_reg) -> Slice25/1
  err_clear_sim23/1 -> delay20/1(sim_1)
  delay20/1(in_reg) -> Slice26/1
  err_clear_sim24/1 -> delay21/1(sim_1)
  delay21/1(in_reg) -> Slice27/1
  err_clear_sim25/1 -> delay22/1(sim_1)
  delay22/1(in_reg) -> Slice28/1
  err_clear_sim26/1 -> delay23/1(sim_1)
  delay23/1(in_reg) -> Slice22/1
  Slice19/1 -> pipeline39/1(d)
  Slice29/1 -> pipeline59/1(d)
  Slice30/1 -> pipeline60/1(d)
  Slice31/1 -> pipeline61/1(d)
  Slice33/1 -> pipeline63/1(d)
  Slice32/1 -> pipeline62/1(d)
  Slice20/1 -> pipeline65/1(d)
  Slice34/1 -> pipeline64/1(d)
  Slice23/1 -> pipeline67/1(d)
  Slice22/1 -> pipeline73/1(d)
  Slice24/1 -> pipeline68/1(d)
  Slice27/1 -> pipeline71/1(d)
  Slice28/1 -> pipeline72/1(d)
  Slice21/1 -> pipeline66/1(d)
  Slice25/1 -> pipeline69/1(d)
  Slice26/1 -> pipeline70/1(d)
  [timing_sync] -> coarse_delay1/1(sync)
  [delay16] -> coarse_delay1/2(delay0)
  [ain16] -> coarse_delay1/3(in0)
  [ain17] -> coarse_delay1/5(in1)
  [delay17] -> coarse_delay1/4(delay1)
  [ain18] -> coarse_delay1/7(in2)
  [ain19] -> coarse_delay1/9(in3)
  [delay18] -> coarse_delay1/6(delay2)
  [delay19] -> coarse_delay1/8(delay3)
  [ain20] -> coarse_delay1/11(in4)
  [ain21] -> coarse_delay1/13(in5)
  [delay21] -> coarse_delay1/12(delay5)
  [delay20] -> coarse_delay1/10(delay4)
  [ain22] -> coarse_delay1/15(in6)
  [ain23] -> coarse_delay1/17(in7)
  [delay22] -> coarse_delay1/14(delay6)
  [delay23] -> coarse_delay1/16(delay7)
  [ain24] -> coarse_delay1/19(in8)
  [ain25] -> coarse_delay1/21(in9)
  [delay25] -> coarse_delay1/20(delay9)
  [delay24] -> coarse_delay1/18(delay8)
  [delay26] -> coarse_delay1/22(delay10)
  [ain31] -> coarse_delay1/33(in15)
  [ain27] -> coarse_delay1/25(in11)
  [ain28] -> coarse_delay1/27(in12)
  [ain26] -> coarse_delay1/23(in10)
  [ain29] -> coarse_delay1/29(in13)
  [ain30] -> coarse_delay1/31(in14)
  [delay27] -> coarse_delay1/24(delay11)
  [delay29] -> coarse_delay1/28(delay13)
  [delay30] -> coarse_delay1/30(delay14)
  [delay28] -> coarse_delay1/26(delay12)
  [delay31] -> coarse_delay1/32(delay15)
  coarse_delay1/2(out0) -> [adc16]
  coarse_delay1/3(out1) -> [adc17]
  coarse_delay1/14(out12) -> [adc28]
  coarse_delay1/4(out2) -> [adc18]
  coarse_delay1/5(out3) -> [adc19]
  coarse_delay1/15(out13) -> [adc29]
  coarse_delay1/6(out4) -> [adc20]
  coarse_delay1/16(out14) -> [adc30]
  coarse_delay1/7(out5) -> [adc21]
  coarse_delay1/17(out15) -> [adc31]
  coarse_delay1/8(out6) -> [adc22]
  coarse_delay1/9(out7) -> [adc23]
  coarse_delay1/10(out8) -> [adc24]
  coarse_delay1/11(out9) -> [adc25]
  coarse_delay1/12(out10) -> [adc26]
  coarse_delay1/13(out11) -> [adc27]
  Logical1/1 -> [sync_to_cdelay]
  pipeline39/1(q) -> [delay16]
  pipeline59/1(q) -> [delay17]
  pipeline51/1(q) -> [delay8]
  pipeline52/1(q) -> [delay9]
  pipeline53/1(q) -> [delay10]
  pipeline54/1(q) -> [delay11]
  pipeline55/1(q) -> [delay12]
  pipeline56/1(q) -> [delay13]
  pipeline57/1(q) -> [delay14]
  pipeline58/1(q) -> [delay15]
  pipeline42/1(q) -> [delay0]
  pipeline43/1(q) -> [delay1]
  pipeline44/1(q) -> [delay2]
  pipeline46/1(q) -> [delay3]
  pipeline47/1(q) -> [delay4]
  pipeline48/1(q) -> [delay5]
  pipeline49/1(q) -> [delay6]
  pipeline50/1(q) -> [delay7]
  adc16x250-8/1(a1) -> ant_remap/1(In1)
  adc16x250-8/2(a2) -> ant_remap/2(In2)
  adc16x250-8/3(a3) -> ant_remap/3(In3)
  adc16x250-8/4(a4) -> ant_remap/4(In4)
  adc16x250-8/5(b1) -> ant_remap/5(In5)
  adc16x250-8/6(b2) -> ant_remap/6(In6)
  adc16x250-8/7(b3) -> ant_remap/7(In7)
  adc16x250-8/8(b4) -> ant_remap/8(In8)
  adc16x250-8/9(c1) -> ant_remap/9(In9)
  adc16x250-8/10(c2) -> ant_remap/10(In10)
  adc16x250-8/11(c3) -> ant_remap/11(In11)
  adc16x250-8/12(c4) -> ant_remap/12(In12)
  adc16x250-8/13(d1) -> ant_remap/13(In13)
  adc16x250-8/14(d2) -> ant_remap/14(In14)
  adc16x250-8/15(d3) -> ant_remap/15(In15)
  adc16x250-8/16(d4) -> ant_remap/16(In16)
  adc16x250-8/17(e1) -> ant_remap/17(In17)
  adc16x250-8/18(e2) -> ant_remap/18(In18)
  adc16x250-8/19(e3) -> ant_remap/19(In19)
  adc16x250-8/20(e4) -> ant_remap/20(In20)
  adc16x250-8/21(f1) -> ant_remap/21(In21)
  adc16x250-8/22(f2) -> ant_remap/22(In22)
  adc16x250-8/23(f3) -> ant_remap/23(In23)
  adc16x250-8/24(f4) -> ant_remap/24(In24)
  adc16x250-8/25(g1) -> ant_remap/25(In25)
  adc16x250-8/26(g2) -> ant_remap/26(In26)
  adc16x250-8/27(g3) -> ant_remap/27(In27)
  adc16x250-8/28(g4) -> ant_remap/28(In28)
  adc16x250-8/29(h1) -> ant_remap/29(In29)
  adc16x250-8/30(h2) -> ant_remap/30(In30)
  adc16x250-8/31(h3) -> ant_remap/31(In31)
  adc16x250-8/32(h4) -> ant_remap/32(In32)
  ant_remap/1(Out1) -> [ain0]
  ant_remap/2(Out2) -> [ain1]
  ant_remap/3(Out3) -> [ain2]
  ant_remap/4(Out4) -> [ain3]
  ant_remap/5(Out5) -> [ain4]
  ant_remap/6(Out6) -> [ain5]
  ant_remap/7(Out7) -> [ain6]
  ant_remap/8(Out8) -> [ain7]
  ant_remap/9(Out9) -> [ain8]
  ant_remap/10(Out10) -> [ain9]
  ant_remap/11(Out11) -> [ain10]
  ant_remap/12(Out12) -> [ain11]
  ant_remap/13(Out13) -> [ain12]
  ant_remap/14(Out14) -> [ain13]
  ant_remap/15(Out15) -> [ain14]
  ant_remap/16(Out16) -> [ain15]
  ant_remap/17(Out17) -> [ain16]
  ant_remap/18(Out18) -> [ain17]
  ant_remap/19(Out19) -> [ain18]
  ant_remap/20(Out20) -> [ain19]
  ant_remap/21(Out21) -> [ain20]
  ant_remap/22(Out22) -> [ain21]
  ant_remap/23(Out23) -> [ain22]
  ant_remap/24(Out24) -> [ain23]
  ant_remap/25(Out25) -> [ain24]
  ant_remap/26(Out26) -> [ain25]
  ant_remap/27(Out27) -> [ain26]
  ant_remap/28(Out28) -> [ain27]
  ant_remap/29(Out29) -> [ain28]
  ant_remap/30(Out30) -> [ain29]
  ant_remap/31(Out31) -> [ain30]
  ant_remap/32(Out32) -> [ain31]
  pipeline68/1(q) -> [delay18]
  pipeline69/1(q) -> [delay19]
  pipeline70/1(q) -> [delay20]
  pipeline71/1(q) -> [delay21]
  pipeline72/1(q) -> [delay22]
  pipeline73/1(q) -> [delay23]
  pipeline60/1(q) -> [delay24]
  pipeline61/1(q) -> [delay25]
  pipeline62/1(q) -> [delay26]
  pipeline63/1(q) -> [delay27]
  pipeline64/1(q) -> [delay28]
  pipeline65/1(q) -> [delay29]
  pipeline66/1(q) -> [delay30]
  pipeline67/1(q) -> [delay31]
